simulink library "blind_cfr_lib"  (Simulink 8.7)
settings: Solver=ode45  StartTime=0.0  StopTime=10.0  RelTol=1e-3
undefined symbols (not defined in the file): AdvDSPBChannelOutDisplay, AdvDSPBDMemDisplay, cfr0_id, cfr_Params, clock_rate, dpoly, dspba_ChannelInVis, dspba_ChannelOutVis, dspba_internal_get_channel_ports, dspba_internal_get_demux_ports, evalAionMaskParam, iq_width, Iter0_Param, latency, primtype, PulsExtention, REG, REG_dut_id_addr, sample_rate, UseDontCare, value, win
libraries: DSPBAPrim x213, blind_cfr_lib x22, DSPBAControl x17, DSPBAModelBus x3, Pipereg_lib x2, CORDIC_lib x1
(part 1 of 3)
settings Model: Creator=nsafari  LastModifiedBy=5g

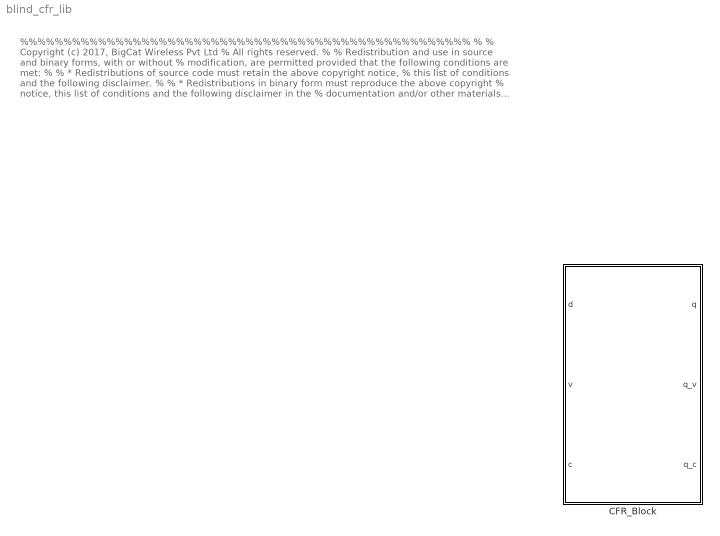
== system blind_cfr_lib ==
  note: %%%%%%%%%%%%%%%%%%%%%%%%%%%%%%%%%%%%%%%%%%%%%%%%%%%%
      |  %
      |  % Copyright (c) 2017, BigCat Wireless Pvt Ltd
      |  % All rights reserved.
      |  %
      |  % Redistribution and use in source and binary forms, with or without
      |  % modification, are permitted provided that the following conditions are met:
      |  %
      |  %     * Redistributions of source code must retain the above copyright notice,
      |  %       this list of conditions and the following disclaimer.
      |  %
      |  %     * Redistributions in binary form must reproduce the above copyright
      |  %       notice, this list of conditions and the following disclaimer in the
      |  %       documentation and/or other materials provided with the distribution.
      |  %
      |  %     * Neither the name of the copyright holder nor the names of its contributors
      |  %       may be used to endorse or promote products derived from this software
      |  %       without specific prior written permission.
      |  %
      |  %
      |  %
      |  % THIS SOFTWARE IS PROVIDED BY THE COPYRIGHT HOLDERS AND CONTRIBUTORS "AS IS"
      |  % AND ANY EXPRESS OR IMPLIED WARRANTIES, INCLUDING, BUT NOT LIMITED TO, THE
      |  % IMPLIED WARRANTIES OF MERCHANTABILITY AND FITNESS FOR A PARTICULAR PURPOSE ARE
      |  % DISCLAIMED. IN NO EVENT SHALL THE COPYRIGHT HOLDER OR CONTRIBUTORS BE LIABLE
      |  % FOR ANY DIRECT, INDIRECT, INCIDENTAL, SPECIAL, EXEMPLARY, OR CONSEQUENTIAL
      |  % DAMAGES (INCLUDING, BUT NOT LIMITED TO, PROCUREMENT OF SUBSTITUTE GOODS OR
      |  % SERVICES; LOSS OF USE, DATA, OR PROFITS; OR BUSINESS INTERRUPTION) HOWEVER
      |  % CAUSED AND ON ANY THEORY OF LIABILITY, WHETHER IN CONTRACT, STRICT LIABILITY,
      |  % OR TORT (INCLUDING NEGLIGENCE OR OTHERWISE) ARISING IN ANY WAY OUT OF THE USE
      |  % OF THIS SOFTWARE, EVEN IF ADVISED OF THE POSSIBILITY OF SUCH DAMAGE.
      |  %
      |   %%%%%%%%%%%%%%%%%%%%%%%%%%%%%%%%%%%%%%%%%%%%%%%%%%%
  CFR_Block : Subsystem  mask(Altera CFR Library Block){clk=clock_rate, sample_rate=sample_rate, block_id=cfr0_id, block_id_addr=REG_dut_id_addr, cfr_Params=cfr_Params, REG=REG, Pipeline_stages=0, ClockMargin=0}
      mask prompts: clk "System clock"; sample_rate "sample rate"; block_id "Unique ID of CFR"; block_id_addr "CFR ID address"; cfr_Params "CFR Configuration Structure"; REG "Register Map"
      mask help:
      | The block has the following parameters:
      |
      | "system clock" - the clock rate CFR module runs.
      |
      | "sample rate" - input signal sampling rate.
      |
      | "Folding Factor" - the number of folding for the module time-sharing;
      | It takes integer values between 1 and floor(system clock / sample rate).
      |
      | "Unique ID of CFR" is a unique numerical integer identifier for the CFR
      | block, this is used once the block is in a larger system to confirm the
      | correct block is being accessed.
      |
      | "CFR ID address" this is the relative address of the "Unique ID of CFR"
      | typically this is zero (at the CFR base address).
      |
      | "CFR Configuration Structure" - an array structure containing the
      | configuration of the CFR block. The length of this parameter specifies the
      | number of CFR core iterations instantiated.
      |
      | "Register Map" a structure containing the register map for CFR block.
      |
      | The settings of the above are exemplified in the setup script of the
      | altera_cfr example design.
      mask init:
      | %setup_cfr_block(iters, Iter_Params, REG, block_id, block_id_addr);
      mask Display:
      | fprintf('BLIND CFR');
      | port_label('input',1,'d');
      | port_label('input',2,'v');
      | port_label('input',3,'c');
      | port_label('output',1,'q');
      | port_label('output',2,'q_v');
      | port_label('output',3,'q_c');

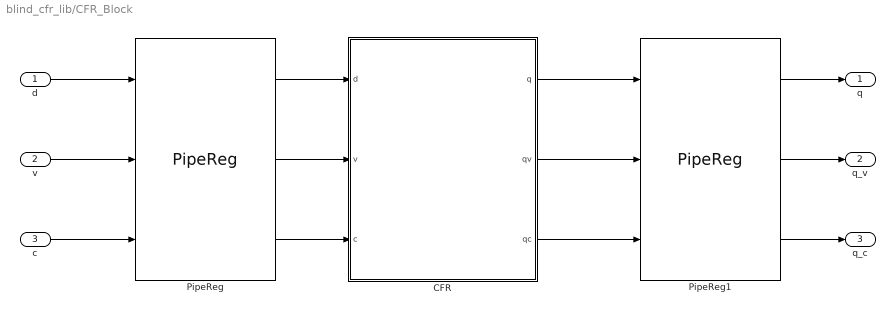
== system blind_cfr_lib/CFR_Block ==
  d : Inport
  v : Inport  Port=2
  c : Inport  Port=3
  CFR : Subsystem
  PipeReg : Pipereg_lib/PipeReg  NPipe=Pipeline_stages  Clock_Margin=ClockMargin
  PipeReg1 : Pipereg_lib/PipeReg  NPipe=Pipeline_stages  Clock_Margin=ClockMargin
  q : Outport
  q_v : Outport  Port=2
  q_c : Outport  Port=3
  wires:
  v/1 -> PipeReg/2
  c/1 -> PipeReg/3
  d/1 -> PipeReg/1
  PipeReg1/2 -> q_v/1
  PipeReg1/3 -> q_c/1
  PipeReg1/1 -> q/1
  PipeReg/2 -> CFR/2(v)
  PipeReg/3 -> CFR/3(c)
  PipeReg/1 -> CFR/1(d)
  CFR/1(q) -> PipeReg1/1
  CFR/2(qv) -> PipeReg1/2
  CFR/3(qc) -> PipeReg1/3

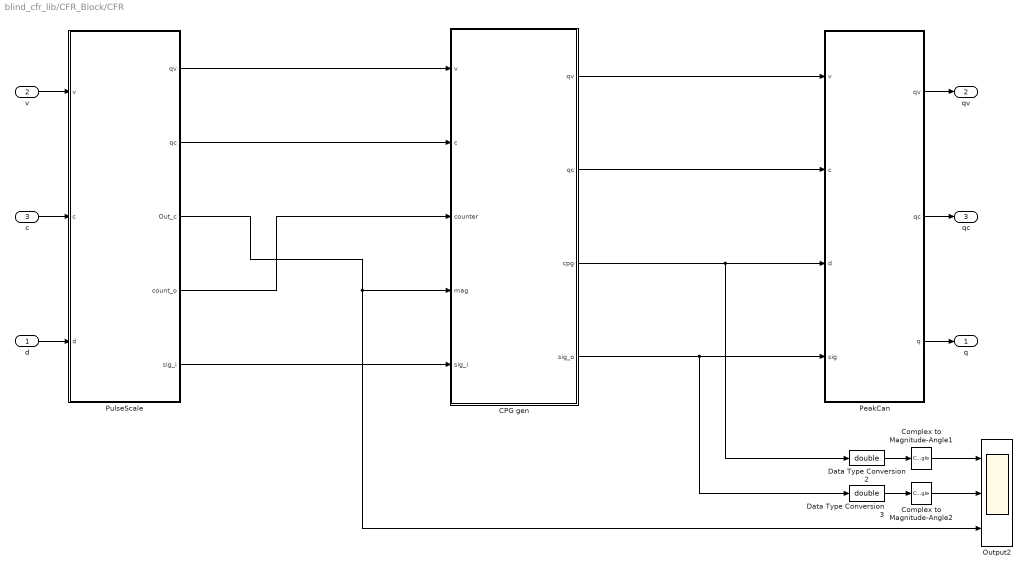
== system blind_cfr_lib/CFR_Block/CFR ==
  d : Inport
  v : Inport  Port=2
  c : Inport  Port=3
  CPG gen : Subsystem
  Complex to Magnitude-Angle1 : ComplexToMagnitudeAngle  Output=Magnitude
  Complex to Magnitude-Angle2 : ComplexToMagnitudeAngle  Output=Magnitude
  Data Type Conversion2 : DataTypeConversion  OutDataTypeStr=double
  Data Type Conversion3 : DataTypeConversion  OutDataTypeStr=double
  Output2 : Scope  NumInputPorts=3
  PeakCan : Subsystem
  PulseScale : Subsystem
  q : Outport
  qv : Outport  Port=2
  qc : Outport  Port=3
  wires:
  v/1 -> PulseScale/1(v)
  c/1 -> PulseScale/2(c)
  PeakCan/1(qv) -> qv/1
  PeakCan/2(qc) -> qc/1
  PeakCan/3(q) -> q/1
  CPG gen/3(cpg) -> Data Type Conversion2/1, PeakCan/3(d)
  CPG gen/4(sig_o) -> Data Type Conversion3/1, PeakCan/4(sig)
  CPG gen/1(qv) -> PeakCan/1(v)
  CPG gen/2(qc) -> PeakCan/2(c)
  PulseScale/1(qv) -> CPG gen/1(v)
  PulseScale/2(qc) -> CPG gen/2(c)
  PulseScale/3(Out_c) -> Output2/3, CPG gen/4(mag)
  PulseScale/4(count_o) -> CPG gen/3(counter)
  Data Type Conversion2/1 -> Complex to Magnitude-Angle1/1
  Complex to Magnitude-Angle1/1 -> Output2/1
  Data Type Conversion3/1 -> Complex to Magnitude-Angle2/1
  Complex to Magnitude-Angle2/1 -> Output2/2
  d/1 -> PulseScale/3(d)
  PulseScale/5(sig_i) -> CPG gen/5(sig_i)

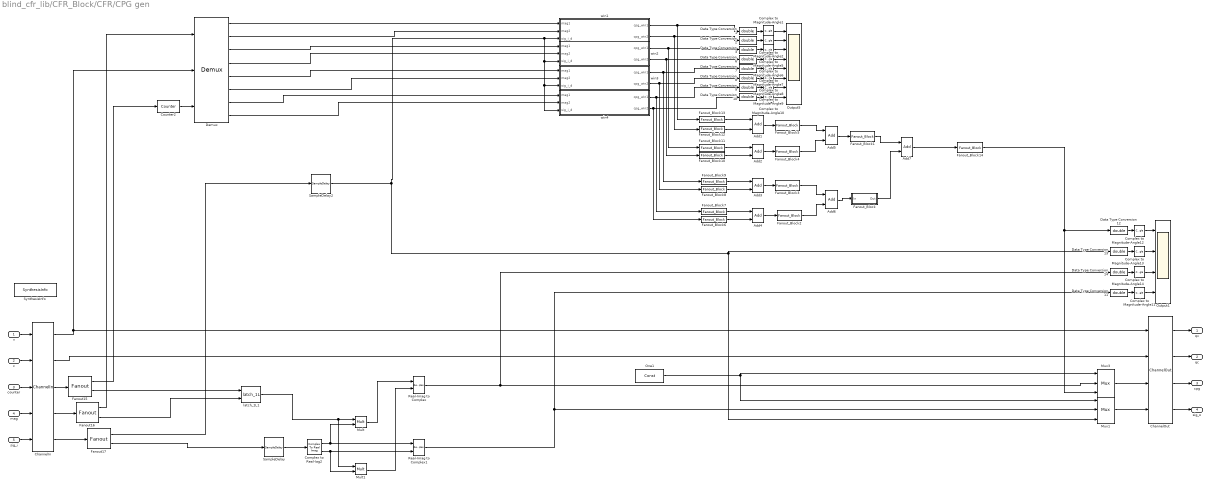
== system blind_cfr_lib/CFR_Block/CFR/CPG gen ==
  v : Inport
  c : Inport  Port=2
  counter : Inport  Port=3
  mag : Inport  Port=4
  sig_i : Inport  Port=5
  Add{1..7} (7 alike) : DSPBAPrim/Add  primtype=add  nInputs=evalAionMaskParam(gcb,'value',1)  nOutputs=1  omode=Inherit via internal rule with word growth  otype=sfix(16)  scale=2^-15  rndmethod=Unbiased  factor=1  satmethod=Symmetric  shift_vec=[0 1 2 -1]  value=2  inPortNames=[' '; ' ';]  outPortNames=[' ']  dspbaimage=dspba_prim.jpg  text=fprintf('+');  style=Optimised  visibilities=1032+2^17+2^18+2^19  genFPC=off  floatRounding=correct  advOptions=[]  version=20130821
  ChannelIn : DSPBAPrim/ChannelIn  primtype=channelin  nInputs=dspba_internal_get_channel_ports(gcb)  nOutputs=dspba_internal_get_channel_ports(gcb)  omode=Inherit via internal rule  otype=sfix(16)  scale=2^-15  rndmethod=Unbiased  factor=1  satmethod=Symmetric  shift_vec=[0 1 2 -1]  value=3  inPortNames=['v'; 'c'; '0'; '1'; '2'; '3'; '4'; '5'; '6'; '7'; '8'; '9'; 'A'; 'B'; 'D'; 'E'; 'F'; 'G'; 'H'; 'I'; 'J'; 'K'; 'L'; 'M'; 'N'; 'O'; 'P'; 'Q'; 'R'; 'S'; 'T'; 'U'; 'W'; 'X'; 'Y'; 'Z']  outPortNames=['v'; 'c'; '0'; '1'; '2'; '3'; '4'; '5'; '6'; '7'; '8'; '9'; 'A'; 'B'; 'D'; 'E'; 'F'; 'G'; 'H'; 'I'; 'J'; 'K'; 'L'; 'M'; 'N'; 'O'; 'P'; 'Q'; 'R'; 'S'; 'T'; 'U'; 'W'; 'X'; 'Y'; 'Z']  dspbaimage=dspba_prim.jpg  text=fprintf('In');  style=Optimised  dataSignals=3  foldingEnabled=off  channels=1  sampleRate=200  packetBeginPresent=off  packetBeginEnabled=off  visibilities=dspba_ChannelInVis(gcb)  latencyCorrection=0  version=20141013
  ChannelOut : DSPBAPrim/ChannelOut  primtype=channelout  nInputs=dspba_internal_get_channel_ports(gcb)  nOutputs=dspba_internal_get_channel_ports(gcb)  omode=Inherit via internal rule  otype=sfix(16)  scale=2^-15  rndmethod=Unbiased  factor=1  satmethod=Symmetric  shift_vec=[0 1 2 -1]  value=2  inPortNames=['v'; 'c'; '0'; '1'; '2'; '3'; '4'; '5'; '6'; '7'; '8'; '9'; 'A'; 'B'; 'D'; 'E'; 'F'; 'G'; 'H'; 'I'; 'J'; 'K'; 'L'; 'M'; 'N'; 'O'; 'P'; 'Q'; 'R'; 'S'; 'T'; 'U'; 'W'; 'X'; 'Y'; 'Z']  outPortNames=['v'; 'c'; '0'; '1'; '2'; '3'; '4'; '5'; '6'; '7'; '8'; '9'; 'A'; 'B'; 'D'; 'E'; 'F'; 'G'; 'H'; 'I'; 'J'; 'K'; 'L'; 'M'; 'N'; 'O'; 'P'; 'Q'; 'R'; 'S'; 'T'; 'U'; 'W'; 'X'; 'Y'; 'Z']  dspbaimage=dspba_prim.jpg  text=fprintf('Out%s', AdvDSPBChannelOutDisplay(latency));  style=Optimised  dataSignals=2  foldingEnabled=off  channels=1  sampleRate=200  packetBeginPresent=off  packetBeginEnabled=off  visibilities=dspba_ChannelOutVis(gcb)  latency=16  latencyCorrection=0  version=20141013
  Complex to Magnitude-Angle{1..2,5..14} (12 alike) : ComplexToMagnitudeAngle  Output=Magnitude
  Complex to Real-Iag2 : ComplexToRealImag
  Counter2 : DSPBAPrim/Counter  primtype=counter  nInputs=1  nOutputs=1  omode=Inherit via internal rule  otype=ufix(16)  scale=2^-0  rndmethod=Unbiased  factor=1  satmethod=Symmetric  shift_vec=[0 1 2 -1]  value=[0 8 1]  inPortNames=[' '; ' ';]  outPortNames=[' ']  dspbaimage=dspba_prim.jpg  text=fprintf('counter\n[%d %d %d]', value(1), value(2), value(3));  style=Optimised  visibilities=8 + 1024  version=20090407
  Data Type Conversion{1..3,6..14} (12 alike) : DataTypeConversion  OutDataTypeStr=double
  Demux : DSPBAPrim/Demux  primtype=demux  nInputs=3  nOutputs=dspba_internal_get_demux_ports(gcb)  omode=Inherit via internal rule  otype=sfix(16)  scale=2^-15  rndmethod=Unbiased  factor=1  satmethod=Symmetric  shift_vec=[0 1 2 3 4 5 6 7]  value=8  inPortNames=['q'; 'v'; 'c']  outPortNames=['c0'; 'c1']  dspbaimage=dspba_prim.jpg  text=fprintf('demux');  style=Optimised  visibilities=1536  version=20100120
  Fanout15 : DSPBAPrim/Fanout  primtype=fanout  nInputs=1  nOutputs=evalAionMaskParam(gcb,'value',1)  omode=Inherit via internal rule  otype=sfix(16)  scale=2^-15  rndmethod=Unbiased  factor=1  satmethod=Symmetric  shift_vec=[0 1 2 -1]  value=2  inPortNames=[' '; ' ';]  outPortNames=[' ']  dspbaimage=dspba_prim.jpg  text=fprintf('fanout')  style=Optimised  visibilities=2^10+2^18  version=20150501  uninit=off
  Fanout16 : DSPBAPrim/Fanout  primtype=fanout  nInputs=1  nOutputs=evalAionMaskParam(gcb,'value',1)  omode=Inherit via internal rule  otype=sfix(16)  scale=2^-15  rndmethod=Unbiased  factor=1  satmethod=Symmetric  shift_vec=[0 1 2 -1]  value=2  inPortNames=[' '; ' ';]  outPortNames=[' ']  dspbaimage=dspba_prim.jpg  text=fprintf('fanout')  style=Optimised  visibilities=2^10+2^18  version=20150501  uninit=off
  Fanout17 : DSPBAPrim/Fanout  primtype=fanout  nInputs=1  nOutputs=evalAionMaskParam(gcb,'value',1)  omode=Inherit via internal rule  otype=sfix(16)  scale=2^-15  rndmethod=Unbiased  factor=1  satmethod=Symmetric  shift_vec=[0 1 2 -1]  value=2  inPortNames=[' '; ' ';]  outPortNames=[' ']  dspbaimage=dspba_prim.jpg  text=fprintf('fanout')  style=Optimised  visibilities=2^10+2^18  version=20150501  uninit=off
  Fanout_Block : Subsystem
  Fanout_Block{1..14} (14 alike) : blind_cfr_lib/CFR_Block/CFR/CPG gen/Fanout_Block
  Mult : DSPBAPrim/Mult  primtype=mult  nInputs=2  nOutputs=1  omode=Inherit via internal rule  otype=sfix(16)  scale=2^-15  rndmethod=Unbiased  factor=1  satmethod=Symmetric  shift_vec=[0 1 2 -1]  value=0  inPortNames=[' '; ' ';]  outPortNames=[' ']  dspbaimage=dspba_prim.jpg  text=fprintf('X');  style=Optimised  visibilities=8+2^18+2^19  floatPrecision=float32_m23  floatRounding=correct  advOptions=[]  version=20130115
  Mult1 : DSPBAPrim/Mult  primtype=mult  nInputs=2  nOutputs=1  omode=Inherit via internal rule  otype=sfix(16)  scale=2^-15  rndmethod=Unbiased  factor=1  satmethod=Symmetric  shift_vec=[0 1 2 -1]  value=0  inPortNames=[' '; ' ';]  outPortNames=[' ']  dspbaimage=dspba_prim.jpg  text=fprintf('X');  style=Optimised  visibilities=8+2^18+2^19  floatPrecision=float32_m23  floatRounding=correct  advOptions=[]  version=20130115
  Mux1 : DSPBAPrim/Mux  primtype=mux  nInputs=evalAionMaskParam(gcb,'value',1)+1  nOutputs=1  omode=Inherit via internal rule  otype=sfix(16)  scale=2^-15  rndmethod=Unbiased  factor=1  satmethod=Symmetric  shift_vec=[0 1 2 -1]  value=2  inPortNames=['s'; 'd0'; 'd1'; 'd2'; 'd3'; 'd4'; 'd5'; 'd6'; 'd7'; 'd8'; 'd9';]  outPortNames=[' ']  dspbaimage=dspba_prim.jpg  text=fprintf('%s', primtype);  style=Optimised  visibilities=1032  version=20131025
  Mux3 : DSPBAPrim/Mux  primtype=mux  nInputs=evalAionMaskParam(gcb,'value',1)+1  nOutputs=1  omode=Inherit via internal rule  otype=sfix(16)  scale=2^-15  rndmethod=Unbiased  factor=1  satmethod=Symmetric  shift_vec=[0 1 2 -1]  value=2  inPortNames=['s'; 'd0'; 'd1'; 'd2'; 'd3'; 'd4'; 'd5'; 'd6'; 'd7'; 'd8'; 'd9';]  outPortNames=[' ']  dspbaimage=dspba_prim.jpg  text=fprintf('%s', primtype);  style=Optimised  visibilities=1032  version=20131025
  One1 : DSPBAPrim/Const  primtype=const  nInputs=0  nOutputs=1  omode=boolean  otype=uint(1)  scale=2^0  rndmethod=Unbiased  factor=1  satmethod=Symmetric  shift_vec=[0 1 2 -1]  value=win_enable  inPortNames=['+'; '+';]  outPortNames=[' ']  dspbaimage=dspba_prim.jpg  text=fprintf('%s', num2str(value));  style=Optimised  visibilities=8 + 1024  floatPrecision=float32_m23  version=20120820
  Output1 : Scope  NumInputPorts=4
  Output5 : Scope  NumInputPorts=8
  Real-Imag to Complex : RealImagToComplex
  Real-Imag to Complex1 : RealImagToComplex
  SampleDelay : DSPBAPrim/SampleDelay  primtype=sampdelay  nInputs=1  nOutputs=1  omode=Inherit via internal rule  otype=uint(16)  scale=2^-0  rndmethod=Unbiased  factor=1  satmethod=Symmetric  shift_vec=[0 1 2 -1]  value=Iter0_Param.pulseLen  inPortNames=[' '; ' ';]  outPortNames=[' ']  dspbaimage=dspba_prim.jpg  text=dpoly(1, eye(1,value+1), 'z')  style=Optimised  visibilities=8 + 1024  flexible=off  slackgroup=0  augmented=0  version=20090407  advOptions=[]
  SampleDelay2 : DSPBAPrim/SampleDelay  primtype=sampdelay  nInputs=1  nOutputs=1  omode=Inherit via internal rule  otype=uint(16)  scale=2^-0  rndmethod=Unbiased  factor=1  satmethod=Symmetric  shift_vec=[0 1 2 -1]  value=Iter0_Param.pulseLen + PulsExtention  inPortNames=[' '; ' ';]  outPortNames=[' ']  dspbaimage=dspba_prim.jpg  text=dpoly(1, eye(1,value+1), 'z')  style=Optimised  visibilities=8 + 1024  flexible=off  slackgroup=0  augmented=0  version=20090407  advOptions=[]
  SynthesisInfo : DSPBAPrim/SynthesisInfo  primtype=synthinfo  nInputs=0  nOutputs=0  omode=Inherit via internal rule  otype=sfix(16)  scale=2^-15  rndmethod=Truncate  factor=1  satmethod=Symmetric  shift_vec=[0 1 2 -1]  value=99  inPortNames=[' '; ' ';]  outPortNames=[' ']  dspbaimage=dspba_prim.jpg  text=fprintf('Style=%s', style);  style=Scheduled  visibilities=32768  constraintInUse=off  constraintRelation=>  constraintLimit=50  bitAccurate=off  version=20150220
  latch_1L1 : DSPBAControl/latch_1L
  win1 : Subsystem
  win2 : Subsystem
  win3 : Subsystem
  win4 : Subsystem
  qv : Outport
  qc : Outport  Port=2
  cpg : Outport  Port=3
  sig_o : Outport  Port=4
  wires:
  Mult/1 -> Real-Imag to Complex/1
  Mult1/1 -> Real-Imag to Complex/2
  Complex to Real-Iag2/2 -> Mult1/2, Real-Imag to Complex1/2
  v/1 -> ChannelIn/1
  c/1 -> ChannelIn/2
  ChannelIn/2 -> ChannelOut/2
  Real-Imag to Complex/1 -> Data Type Conversion14/1, Mux3/2
  ChannelOut/1 -> qv/1
  ChannelOut/2 -> qc/1
  counter/1 -> ChannelIn/3
  mag/1 -> ChannelIn/4
  ChannelOut/3 -> cpg/1
  ChannelOut/4 -> sig_o/1
  Complex to Real-Iag2/1 -> Mult/2, Real-Imag to Complex1/1
  Real-Imag to Complex1/1 -> Mux1/2, Data Type Conversion11/1
  sig_i/1 -> ChannelIn/5
  latch_1L1/1 -> Mult1/1, Mult/1
  ChannelIn/1 -> Demux/2, ChannelOut/1
  SampleDelay/1 -> Complex to Real-Iag2/1
  Counter2/1 -> Demux/3
  Data Type Conversion1/1 -> Complex to Magnitude-Angle1/1
  Complex to Magnitude-Angle1/1 -> Output5/1
  Data Type Conversion2/1 -> Complex to Magnitude-Angle2/1
  Complex to Magnitude-Angle2/1 -> Output5/2
  Demux/1 -> win1/1(mag1)
  Demux/2 -> win1/2(mag2)
  SampleDelay2/1 -> win1/3(sig_i_d), win2/3(sig_i_d), win4/3(sig_i_d), win3/3(sig_i_d), Mux1/3, Data Type Conversion13/1
  win1/1(cpg_win1) -> Fanout_Block13/1, Data Type Conversion1/1
  win1/2(cpg_win2) -> Fanout_Block12/1, Data Type Conversion2/1
  Demux/3 -> win2/1(mag1)
  Demux/4 -> win2/2(mag2)
  Data Type Conversion3/1 -> Complex to Magnitude-Angle5/1
  Complex to Magnitude-Angle5/1 -> Output5/3
  Data Type Conversion6/1 -> Complex to Magnitude-Angle6/1
  Complex to Magnitude-Angle6/1 -> Output5/4
  Data Type Conversion7/1 -> Complex to Magnitude-Angle7/1
  Complex to Magnitude-Angle7/1 -> Output5/5
  Data Type Conversion8/1 -> Complex to Magnitude-Angle8/1
  Complex to Magnitude-Angle8/1 -> Output5/6
  Data Type Conversion9/1 -> Complex to Magnitude-Angle9/1
  Complex to Magnitude-Angle9/1 -> Output5/7
  Data Type Conversion10/1 -> Complex to Magnitude-Angle10/1
  Complex to Magnitude-Angle10/1 -> Output5/8
  win2/1(cpg_win1) -> Fanout_Block11/1, Data Type Conversion3/1
  win2/2(cpg_win2) -> Fanout_Block10/1, Data Type Conversion6/1
  Demux/5 -> win3/1(mag1)
  Demux/6 -> win3/2(mag2)
  Demux/7 -> win4/1(mag1)
  Demux/8 -> win4/2(mag2)
  win3/1(cpg_win1) -> Fanout_Block9/1, Data Type Conversion7/1
  win3/2(cpg_win2) -> Fanout_Block8/1, Data Type Conversion8/1
  win4/1(cpg_win1) -> Fanout_Block7/1, Data Type Conversion9/1
  win4/2(cpg_win2) -> Fanout_Block6/1, Data Type Conversion10/1
  Data Type Conversion12/1 -> Complex to Magnitude-Angle12/1
  Complex to Magnitude-Angle12/1 -> Output1/1
  Data Type Conversion13/1 -> Complex to Magnitude-Angle13/1
  Complex to Magnitude-Angle13/1 -> Output1/2
  Data Type Conversion14/1 -> Complex to Magnitude-Angle14/1
  Complex to Magnitude-Angle14/1 -> Output1/3
  Data Type Conversion11/1 -> Complex to Magnitude-Angle11/1
  Complex to Magnitude-Angle11/1 -> Output1/4
  One1/1 -> Mux1/1, Mux3/1
  Mux3/1 -> ChannelOut/3
  Mux1/1 -> ChannelOut/4
  Fanout_Block13/1 -> Add1/1
  Fanout_Block12/1 -> Add1/2
  Fanout_Block14/1 -> Data Type Conversion12/1, Mux3/3
  Fanout_Block11/1 -> Add2/1
  Fanout_Block10/1 -> Add2/2
  Fanout_Block9/1 -> Add3/1
  Fanout_Block8/1 -> Add3/2
  Fanout_Block7/1 -> Add4/1
  Add1/1 -> Fanout_Block5/1
  Add4/1 -> Fanout_Block2/1
  Add3/1 -> Fanout_Block3/1
  Add2/1 -> Fanout_Block4/1
  Fanout_Block5/1 -> Add5/1
  Fanout_Block4/1 -> Add5/2
  Fanout_Block3/1 -> Add6/1
  Fanout_Block2/1 -> Add6/2
  Add5/1 -> Fanout_Block1/1
  Fanout_Block1/1 -> Add7/1
  Add7/1 -> Fanout_Block14/1
  ChannelIn/3 -> Fanout15/1
  Fanout15/2 -> latch_1L1/1
  Fanout15/1 -> Counter2/1
  ChannelIn/4 -> Fanout16/1
  Fanout16/1 -> Demux/1
  Fanout16/2 -> latch_1L1/2
  ChannelIn/5 -> Fanout17/1
  Fanout17/2 -> SampleDelay/1
  Fanout17/1 -> SampleDelay2/1
  Add6/1 -> Fanout_Block/1(In)
  Fanout_Block/1(Out) -> Add7/2
  Fanout_Block6/1 -> Add4/2

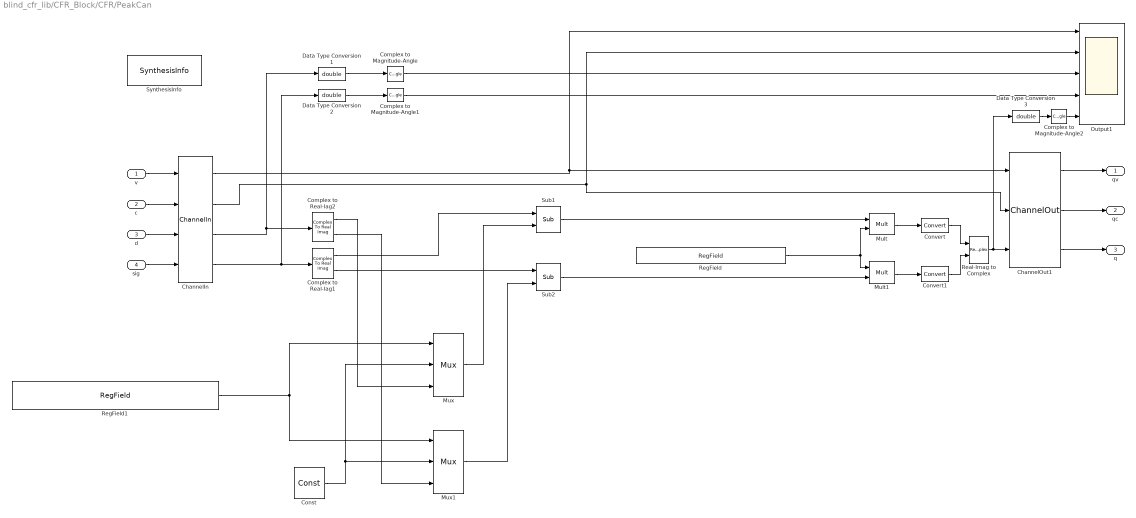
== system blind_cfr_lib/CFR_Block/CFR/PeakCan ==
  v : Inport
  c : Inport  Port=2
  d : Inport  Port=3
  sig : Inport  Port=4
  ChannelIn : DSPBAPrim/ChannelIn  primtype=channelin  nInputs=dspba_internal_get_channel_ports(gcb)  nOutputs=dspba_internal_get_channel_ports(gcb)  omode=Inherit via internal rule  otype=sfix(16)  scale=2^-15  rndmethod=Unbiased  factor=1  satmethod=Symmetric  shift_vec=[0 1 2 -1]  value=2  inPortNames=['v'; 'c'; '0'; '1'; '2'; '3'; '4'; '5'; '6'; '7'; '8'; '9'; 'A'; 'B'; 'D'; 'E'; 'F'; 'G'; 'H'; 'I'; 'J'; 'K'; 'L'; 'M'; 'N'; 'O'; 'P'; 'Q'; 'R'; 'S'; 'T'; 'U'; 'W'; 'X'; 'Y'; 'Z']  outPortNames=['v'; 'c'; '0'; '1'; '2'; '3'; '4'; '5'; '6'; '7'; '8'; '9'; 'A'; 'B'; 'D'; 'E'; 'F'; 'G'; 'H'; 'I'; 'J'; 'K'; 'L'; 'M'; 'N'; 'O'; 'P'; 'Q'; 'R'; 'S'; 'T'; 'U'; 'W'; 'X'; 'Y'; 'Z']  dspbaimage=dspba_prim.jpg  text=fprintf('In');  style=Optimised  dataSignals=2  foldingEnabled=off  channels=1  sampleRate=200  packetBeginPresent=off  packetBeginEnabled=off  visibilities=dspba_ChannelInVis(gcb)  latencyCorrection=0  version=20141013
  ChannelOut1 : DSPBAPrim/ChannelOut  primtype=channelout  nInputs=dspba_internal_get_channel_ports(gcb)  nOutputs=dspba_internal_get_channel_ports(gcb)  omode=Inherit via internal rule  otype=sfix(16)  scale=2^-15  rndmethod=Unbiased  factor=1  satmethod=Symmetric  shift_vec=[0 1 2 -1]  value=1  inPortNames=['v'; 'c'; '0'; '1'; '2'; '3'; '4'; '5'; '6'; '7'; '8'; '9'; 'A'; 'B'; 'D'; 'E'; 'F'; 'G'; 'H'; 'I'; 'J'; 'K'; 'L'; 'M'; 'N'; 'O'; 'P'; 'Q'; 'R'; 'S'; 'T'; 'U'; 'W'; 'X'; 'Y'; 'Z']  outPortNames=['v'; 'c'; '0'; '1'; '2'; '3'; '4'; '5'; '6'; '7'; '8'; '9'; 'A'; 'B'; 'D'; 'E'; 'F'; 'G'; 'H'; 'I'; 'J'; 'K'; 'L'; 'M'; 'N'; 'O'; 'P'; 'Q'; 'R'; 'S'; 'T'; 'U'; 'W'; 'X'; 'Y'; 'Z']  dspbaimage=dspba_prim.jpg  text=fprintf('Out%s', AdvDSPBChannelOutDisplay(latency));  style=Optimised  dataSignals=1  foldingEnabled=off  channels=1  sampleRate=200  packetBeginPresent=off  packetBeginEnabled=off  visibilities=dspba_ChannelOutVis(gcb)  latency=12  latencyCorrection=0  version=20141013
  Complex to Magnitude-Angle : ComplexToMagnitudeAngle  Output=Magnitude
  Complex to Magnitude-Angle1 : ComplexToMagnitudeAngle  Output=Magnitude
  Complex to Magnitude-Angle2 : ComplexToMagnitudeAngle  Output=Magnitude
  Complex to Real-Iag1 : ComplexToRealImag
  Complex to Real-Iag2 : ComplexToRealImag
  Const : DSPBAPrim/Const  primtype=const  nInputs=0  nOutputs=1  omode=Inherit via internal rule  otype=sfix(16)  scale=2^-15  rndmethod=Unbiased  factor=1  satmethod=Symmetric  shift_vec=[0 1 2 -1]  value=0  inPortNames=['+'; '+';]  outPortNames=[' ']  dspbaimage=dspba_prim.jpg  text=fprintf('%s', num2str(value));  style=Optimised  visibilities=8 + 1024  floatPrecision=float32_m23  version=20120820
  Convert : DSPBAPrim/Convert  primtype=convert  nInputs=1  nOutputs=1  omode=Specify via dialog  otype=sfix(16)  scale=2^-15  rndmethod=Unbiased  factor=1  satmethod=None  shift_vec=[0 1 2 -1]  value=round([0:255]/17)  inPortNames=[' '; ' ';]  outPortNames=[' '; 'c']  dspbaimage=dspba_prim.jpg  text=fprintf('convert');  style=Optimised  visibilities=8+64+256+2^17  clipdetect=off  floatPrecision=float32_m23  advOptions=[]  version=20130211
  Convert1 : DSPBAPrim/Convert  primtype=convert  nInputs=1  nOutputs=1  omode=Specify via dialog  otype=sfix(16)  scale=2^-15  rndmethod=Unbiased  factor=1  satmethod=None  shift_vec=[0 1 2 -1]  value=round([0:255]/17)  inPortNames=[' '; ' ';]  outPortNames=[' '; 'c']  dspbaimage=dspba_prim.jpg  text=fprintf('convert');  style=Optimised  visibilities=8+64+256+2^17  clipdetect=off  floatPrecision=float32_m23  advOptions=[]  version=20130211
  Data Type Conversion1 : DataTypeConversion  OutDataTypeStr=double
  Data Type Conversion2 : DataTypeConversion  OutDataTypeStr=double
  Data Type Conversion3 : DataTypeConversion  OutDataTypeStr=double
  Mult : DSPBAPrim/Mult  primtype=mult  nInputs=2  nOutputs=1  omode=Inherit via internal rule  otype=sfix(16)  scale=2^-15  rndmethod=Unbiased  factor=1  satmethod=Symmetric  shift_vec=[0 1 2 -1]  value=0  inPortNames=[' '; ' ';]  outPortNames=[' ']  dspbaimage=dspba_prim.jpg  text=fprintf('X');  style=Optimised  visibilities=8+2^18+2^19  floatPrecision=float32_m23  floatRounding=correct  advOptions=[]  version=20130115
  Mult1 : DSPBAPrim/Mult  primtype=mult  nInputs=2  nOutputs=1  omode=Inherit via internal rule  otype=sfix(16)  scale=2^-15  rndmethod=Unbiased  factor=1  satmethod=Symmetric  shift_vec=[0 1 2 -1]  value=0  inPortNames=[' '; ' ';]  outPortNames=[' ']  dspbaimage=dspba_prim.jpg  text=fprintf('X');  style=Optimised  visibilities=8+2^18+2^19  floatPrecision=float32_m23  floatRounding=correct  advOptions=[]  version=20130115
  Mux : DSPBAPrim/Mux  primtype=mux  nInputs=evalAionMaskParam(gcb,'value',1)+1  nOutputs=1  omode=Inherit via internal rule  otype=sfix(16)  scale=2^-15  rndmethod=Unbiased  factor=1  satmethod=Symmetric  shift_vec=[0 1 2 -1]  value=2  inPortNames=['s '; 'd0'; 'd1'; 'd2'; 'd3'; 'd4'; 'd5'; 'd6'; 'd7'; 'd8'; 'd9';]  outPortNames=[' ']  dspbaimage=dspba_prim.jpg  text=fprintf('%s', primtype);  style=Optimised  visibilities=1032  version=20131025
  Mux1 : DSPBAPrim/Mux  primtype=mux  nInputs=evalAionMaskParam(gcb,'value',1)+1  nOutputs=1  omode=Inherit via internal rule  otype=sfix(16)  scale=2^-15  rndmethod=Unbiased  factor=1  satmethod=Symmetric  shift_vec=[0 1 2 -1]  value=2  inPortNames=['s '; 'd0'; 'd1'; 'd2'; 'd3'; 'd4'; 'd5'; 'd6'; 'd7'; 'd8'; 'd9';]  outPortNames=[' ']  dspbaimage=dspba_prim.jpg  text=fprintf('%s', primtype);  style=Optimised  visibilities=1032  version=20131025
  Output1 : Scope  NumInputPorts=5
  Real-Imag to Complex : RealImagToComplex
  RegField : DSPBAModelBus/RegField  reg_name=cfr_Params.BaseAddr + REG.Scaling  reg_rwmode=Read/Write  reg_msb=15  reg_lsb=0  reg_mode=Specify via dialog  reg_type=ufix(16)  reg_scale=2^-14  reg_init=cfr_Params.Scaling  reg_desc=Scaling value  reg_modal=off  reg_desc0=0  reg_desc1=0  reg_desc2=0  reg_desc3=0  reg_desc4=0  reg_desc5=0  reg_desc6=0  reg_desc7=0  SampleTime=1  version=20090407
  RegField1 : DSPBAModelBus/RegField  reg_name=cfr_Params.BaseAddr + REG.Enable  reg_rwmode=Read/Write  reg_msb=0  reg_lsb=0  reg_mode=Specify via dialog  reg_type=ufix(1)  reg_scale=2^0  reg_init=cfr_Params.Enable  reg_desc=Enable CFR  reg_modal=off  reg_desc0=0  reg_desc1=0  reg_desc2=0  reg_desc3=0  reg_desc4=0  reg_desc5=0  reg_desc6=0  reg_desc7=0  SampleTime=1  version=20090407
  Sub1 : DSPBAPrim/Sub  primtype=sub  nInputs=2  nOutputs=1  omode=Inherit via internal rule  otype=sfix(16)  scale=2^-15  rndmethod=Unbiased  factor=1  satmethod=Symmetric  shift_vec=[0 1 2 -1]  value=0  inPortNames=['+'; '-';]  outPortNames=[' ']  dspbaimage=dspba_prim.jpg  text=fprintf('-');  style=Optimised  visibilities=8  floatRounding=correct  advOptions=[]  version=20130115
  Sub2 : DSPBAPrim/Sub  primtype=sub  nInputs=2  nOutputs=1  omode=Inherit via internal rule  otype=sfix(16)  scale=2^-15  rndmethod=Unbiased  factor=1  satmethod=Symmetric  shift_vec=[0 1 2 -1]  value=0  inPortNames=['+'; '-';]  outPortNames=[' ']  dspbaimage=dspba_prim.jpg  text=fprintf('-');  style=Optimised  visibilities=8  floatRounding=correct  advOptions=[]  version=20130115
  SynthesisInfo : DSPBAPrim/SynthesisInfo  primtype=synthinfo  nInputs=0  nOutputs=0  omode=Inherit via internal rule  otype=sfix(16)  scale=2^-15  rndmethod=Truncate  factor=1  satmethod=Symmetric  shift_vec=[0 1 2 -1]  value=99  inPortNames=[' '; ' ';]  outPortNames=[' ']  dspbaimage=dspba_prim.jpg  text=fprintf('Style=%s', style);  style=Scheduled  visibilities=32768  constraintInUse=off  constraintRelation=>  constraintLimit=20  bitAccurate=off  version=20150220
  qv : Outport
  qc : Outport  Port=2
  q : Outport  Port=3
  wires:
  Data Type Conversion1/1 -> Complex to Magnitude-Angle/1
  Complex to Magnitude-Angle/1 -> Output1/3
  ChannelIn/3 -> Data Type Conversion1/1, Complex to Real-Iag2/1
  Data Type Conversion2/1 -> Complex to Magnitude-Angle1/1
  Complex to Magnitude-Angle1/1 -> Output1/4
  Real-Imag to Complex/1 -> Data Type Conversion3/1, ChannelOut1/3
  Complex to Real-Iag1/1 -> Sub1/1
  Complex to Real-Iag1/2 -> Sub2/1
  ChannelIn/1 -> Output1/1, ChannelOut1/1
  ChannelIn/2 -> ChannelOut1/2, Output1/2
  v/1 -> ChannelIn/1
  d/1 -> ChannelIn/3
  c/1 -> ChannelIn/2
  sig/1 -> ChannelIn/4
  ChannelOut1/1 -> qv/1
  ChannelOut1/2 -> qc/1
  ChannelOut1/3 -> q/1
  ChannelIn/4 -> Complex to Real-Iag1/1, Data Type Conversion2/1
  RegField/1 -> Mult/2, Mult1/1
  Mult/1 -> Convert/1
  Mult1/1 -> Convert1/1
  Sub1/1 -> Mult/1
  Sub2/1 -> Mult1/2
  Convert/1 -> Real-Imag to Complex/1
  Convert1/1 -> Real-Imag to Complex/2
  Data Type Conversion3/1 -> Complex to Magnitude-Angle2/1
  Complex to Magnitude-Angle2/1 -> Output1/5
  RegField1/1 -> Mux/1, Mux1/1
  Complex to Real-Iag2/1 -> Mux/3
  Complex to Real-Iag2/2 -> Mux1/3
  Mux/1 -> Sub1/2
  Mux1/1 -> Sub2/2
  Const/1 -> Mux/2, Mux1/2

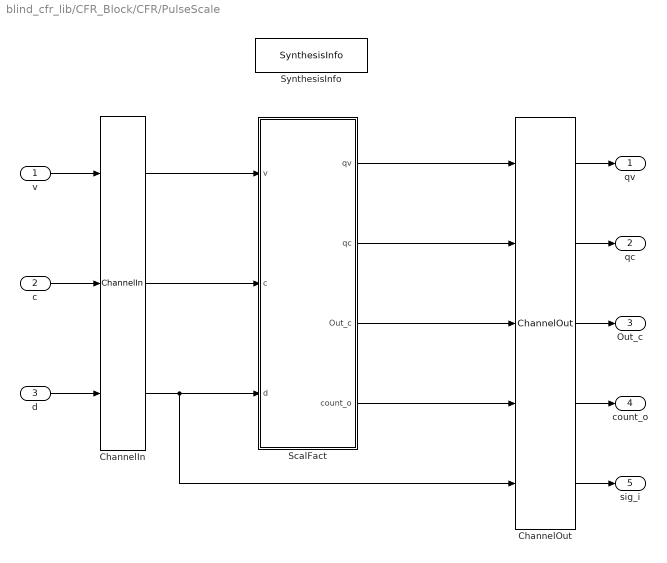
== system blind_cfr_lib/CFR_Block/CFR/PulseScale ==
  v : Inport
  c : Inport  Port=2
  d : Inport  Port=3
  ChannelIn : DSPBAPrim/ChannelIn  primtype=channelin  nInputs=dspba_internal_get_channel_ports(gcb)  nOutputs=dspba_internal_get_channel_ports(gcb)  omode=Inherit via internal rule  otype=sfix(16)  scale=2^-15  rndmethod=Unbiased  factor=1  satmethod=Symmetric  shift_vec=[0 1 2 -1]  value=1  inPortNames=['v'; 'c'; '0'; '1'; '2'; '3'; '4'; '5'; '6'; '7'; '8'; '9'; 'A'; 'B'; 'D'; 'E'; 'F'; 'G'; 'H'; 'I'; 'J'; 'K'; 'L'; 'M'; 'N'; 'O'; 'P'; 'Q'; 'R'; 'S'; 'T'; 'U'; 'W'; 'X'; 'Y'; 'Z']  outPortNames=['v'; 'c'; '0'; '1'; '2'; '3'; '4'; '5'; '6'; '7'; '8'; '9'; 'A'; 'B'; 'D'; 'E'; 'F'; 'G'; 'H'; 'I'; 'J'; 'K'; 'L'; 'M'; 'N'; 'O'; 'P'; 'Q'; 'R'; 'S'; 'T'; 'U'; 'W'; 'X'; 'Y'; 'Z']  dspbaimage=dspba_prim.jpg  text=fprintf('In');  style=Optimised  dataSignals=1  foldingEnabled=off  channels=1  sampleRate=200  packetBeginPresent=off  packetBeginEnabled=off  visibilities=dspba_ChannelInVis(gcb)  latencyCorrection=0  version=20141013
  ChannelOut : DSPBAPrim/ChannelOut  primtype=channelout  nInputs=dspba_internal_get_channel_ports(gcb)  nOutputs=dspba_internal_get_channel_ports(gcb)  omode=Inherit via internal rule  otype=sfix(16)  scale=2^-15  rndmethod=Unbiased  factor=1  satmethod=Symmetric  shift_vec=[0 1 2 -1]  value=3  inPortNames=['v'; 'c'; '0'; '1'; '2'; '3'; '4'; '5'; '6'; '7'; '8'; '9'; 'A'; 'B'; 'D'; 'E'; 'F'; 'G'; 'H'; 'I'; 'J'; 'K'; 'L'; 'M'; 'N'; 'O'; 'P'; 'Q'; 'R'; 'S'; 'T'; 'U'; 'W'; 'X'; 'Y'; 'Z']  outPortNames=['v'; 'c'; '0'; '1'; '2'; '3'; '4'; '5'; '6'; '7'; '8'; '9'; 'A'; 'B'; 'D'; 'E'; 'F'; 'G'; 'H'; 'I'; 'J'; 'K'; 'L'; 'M'; 'N'; 'O'; 'P'; 'Q'; 'R'; 'S'; 'T'; 'U'; 'W'; 'X'; 'Y'; 'Z']  dspbaimage=dspba_prim.jpg  text=fprintf('Out%s', AdvDSPBChannelOutDisplay(latency));  style=Optimised  dataSignals=3  foldingEnabled=off  channels=1  sampleRate=200  packetBeginPresent=off  packetBeginEnabled=off  visibilities=dspba_ChannelOutVis(gcb)  latency=24  latencyCorrection=0  version=20141013
  ScalFact : Subsystem
  SynthesisInfo : DSPBAPrim/SynthesisInfo  primtype=synthinfo  nInputs=0  nOutputs=0  omode=Inherit via internal rule  otype=sfix(16)  scale=2^-15  rndmethod=Truncate  factor=1  satmethod=Symmetric  shift_vec=[0 1 2 -1]  value=99  inPortNames=[' '; ' ';]  outPortNames=[' ']  dspbaimage=dspba_prim.jpg  text=fprintf('Style=%s', style);  style=Scheduled  visibilities=32768  constraintInUse=off  constraintRelation=>  constraintLimit=50  bitAccurate=off  version=20150220
  qv : Outport
  qc : Outport  Port=2
  Out_c : Outport  Port=3
  count_o : Outport  Port=4
  sig_i : Outport  Port=5
  wires:
  v/1 -> ChannelIn/1
  c/1 -> ChannelIn/2
  ScalFact/1(qv) -> ChannelOut/1
  ScalFact/2(qc) -> ChannelOut/2
  ScalFact/3(Out_c) -> ChannelOut/3
  d/1 -> ChannelIn/3
  ChannelIn/1 -> ScalFact/1(v)
  ChannelIn/2 -> ScalFact/2(c)
  ChannelIn/3 -> ScalFact/3(d), ChannelOut/5
  ChannelOut/1 -> qv/1
  ChannelOut/2 -> qc/1
  ChannelOut/3 -> Out_c/1
  ScalFact/4(count_o) -> ChannelOut/4
  ChannelOut/4 -> count_o/1
  ChannelOut/5 -> sig_i/1

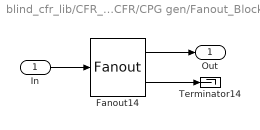
== system blind_cfr_lib/CFR_Block/CFR/CPG gen/Fanout_Block ==
  In : Inport
  Fanout14 : DSPBAPrim/Fanout  primtype=fanout  nInputs=1  nOutputs=evalAionMaskParam(gcb,'value',1)  omode=Inherit via internal rule  otype=sfix(16)  scale=2^-15  rndmethod=Unbiased  factor=1  satmethod=Symmetric  shift_vec=[0 1 2 -1]  value=2  inPortNames=[' '; ' ';]  outPortNames=[' ']  dspbaimage=dspba_prim.jpg  text=fprintf('fanout')  style=Optimised  visibilities=2^10+2^18  version=20150501  uninit=off
  Terminator14 : Terminator
  Out : Outport
  wires:
  Fanout14/2 -> Terminator14/1
  In/1 -> Fanout14/1
  Fanout14/1 -> Out/1

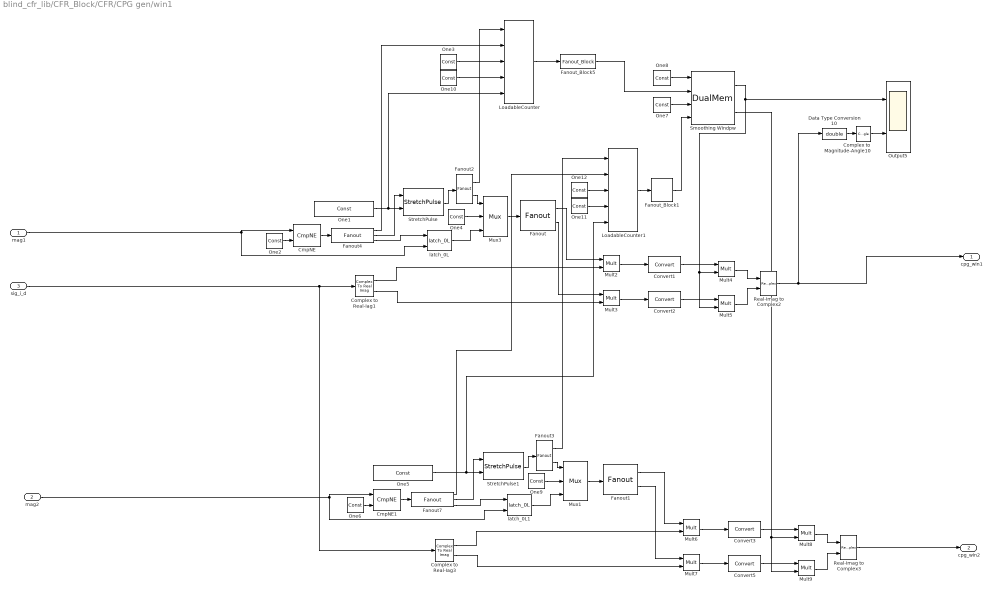
== system blind_cfr_lib/CFR_Block/CFR/CPG gen/win1 ==
  mag1 : Inport
  mag2 : Inport  Port=2
  sig_i_d : Inport  Port=3
  CmpNE : DSPBAPrim/CmpNE  primtype=cmpne  nInputs=2  nOutputs=1  omode=boolean  otype=sfix(16)  scale=2^-15  rndmethod=Unbiased  factor=1  satmethod=Symmetric  shift_vec=[0 1 2 -1]  value=0  inPortNames=[' '; ' ';]  outPortNames=[' ']  dspbaimage=dspba_prim.jpg  text=fprintf('~=');  style=Optimised  visibilities=0  advOptions=[]  version=20130117
  CmpNE1 : DSPBAPrim/CmpNE  primtype=cmpne  nInputs=2  nOutputs=1  omode=boolean  otype=sfix(16)  scale=2^-15  rndmethod=Unbiased  factor=1  satmethod=Symmetric  shift_vec=[0 1 2 -1]  value=0  inPortNames=[' '; ' ';]  outPortNames=[' ']  dspbaimage=dspba_prim.jpg  text=fprintf('~=');  style=Optimised  visibilities=0  advOptions=[]  version=20130117
  Complex to Magnitude-Angle10 : ComplexToMagnitudeAngle  Output=Magnitude
  Complex to Real-Iag1 : ComplexToRealImag
  Complex to Real-Iag3 : ComplexToRealImag
  Convert{1..3,5} (4 alike) : DSPBAPrim/Convert  primtype=convert  nInputs=1  nOutputs=1  omode=Specify via dialog  otype=sfix(16)  scale=2^-(15)  rndmethod=Unbiased  factor=1  satmethod=None  shift_vec=[0 1 2 -1]  value=round([0:255]/17)  inPortNames=[' '; ' ';]  outPortNames=[' '; 'c']  dspbaimage=dspba_prim.jpg  text=fprintf('convert');  style=Optimised  visibilities=8+64+256  clipdetect=off  floatPrecision=float32_m23  advOptions=[]  version=20130211
  Data Type Conversion10 : DataTypeConversion  OutDataTypeStr=double
  Fanout{,1..3} (4 alike) : DSPBAPrim/Fanout  primtype=fanout  nInputs=1  nOutputs=evalAionMaskParam(gcb,'value',1)  omode=Inherit via internal rule  otype=sfix(16)  scale=2^-15  rndmethod=Unbiased  factor=1  satmethod=Symmetric  shift_vec=[0 1 2 -1]  value=2  inPortNames=[' '; ' ';]  outPortNames=[' ']  dspbaimage=dspba_prim.jpg  text=fprintf('fanout')  style=Optimised  visibilities=2^10+2^18  version=20150501  uninit=off
  Fanout4 : DSPBAPrim/Fanout  primtype=fanout  nInputs=1  nOutputs=evalAionMaskParam(gcb,'value',1)  omode=Inherit via internal rule  otype=sfix(16)  scale=2^-15  rndmethod=Unbiased  factor=1  satmethod=Symmetric  shift_vec=[0 1 2 -1]  value=3  inPortNames=[' '; ' ';]  outPortNames=[' ']  dspbaimage=dspba_prim.jpg  text=fprintf('fanout')  style=Optimised  visibilities=2^10+2^18  version=20150501  uninit=off
  Fanout7 : DSPBAPrim/Fanout  primtype=fanout  nInputs=1  nOutputs=evalAionMaskParam(gcb,'value',1)  omode=Inherit via internal rule  otype=sfix(16)  scale=2^-15  rndmethod=Unbiased  factor=1  satmethod=Symmetric  shift_vec=[0 1 2 -1]  value=3  inPortNames=[' '; ' ';]  outPortNames=[' ']  dspbaimage=dspba_prim.jpg  text=fprintf('fanout')  style=Optimised  visibilities=2^10+2^18  version=20150501  uninit=off
  Fanout_Block1 : blind_cfr_lib/CFR_Block/CFR/CPG gen/Fanout_Block
  Fanout_Block5 : blind_cfr_lib/CFR_Block/CFR/CPG gen/Fanout_Block
  LoadableCounter : DSPBAPrim/LoadableCounter  primtype=loadablecounter  nInputs=5  nOutputs=1  omode=Inherit via internal rule  otype=ufix(16)  scale=2^-0  rndmethod=Unbiased  factor=1  satmethod=Symmetric  shift_vec=[0 1 2 -1]  value=[0 length(win) 1]  inPortNames=['en';'ld';'i ';'s ';'m ']  outPortNames=[' ']  dspbaimage=dspba_prim.jpg  text=fprintf('loadable\ncounter\n[%d %d %d]', value(1), value(2), value(3));  style=Optimised  visibilities=8 + 1024  version=20090407
  LoadableCounter1 : DSPBAPrim/LoadableCounter  primtype=loadablecounter  nInputs=5  nOutputs=1  omode=Inherit via internal rule  otype=ufix(16)  scale=2^-0  rndmethod=Unbiased  factor=1  satmethod=Symmetric  shift_vec=[0 1 2 -1]  value=[0 length(win) 1]  inPortNames=['en';'ld';'i ';'s ';'m ']  outPortNames=[' ']  dspbaimage=dspba_prim.jpg  text=fprintf('loadable\ncounter\n[%d %d %d]', value(1), value(2), value(3));  style=Optimised  visibilities=8 + 1024  version=20090407
  Mult{2..9} (8 alike) : DSPBAPrim/Mult  primtype=mult  nInputs=2  nOutputs=1  omode=Inherit via internal rule  otype=sfix(16)  scale=2^-15  rndmethod=Unbiased  factor=1  satmethod=Symmetric  shift_vec=[0 1 2 -1]  value=0  inPortNames=[' '; ' ';]  outPortNames=[' ']  dspbaimage=dspba_prim.jpg  text=fprintf('X');  style=Optimised  visibilities=8+2^18+2^19  floatPrecision=float32_m23  floatRounding=correct  advOptions=[]  version=20130115
  Mux1 : DSPBAPrim/Mux  primtype=mux  nInputs=evalAionMaskParam(gcb,'value',1)+1  nOutputs=1  omode=Inherit via internal rule  otype=sfix(16)  scale=2^-15  rndmethod=Unbiased  factor=1  satmethod=Symmetric  shift_vec=[0 1 2 -1]  value=2  inPortNames=['s'; 'd0'; 'd1'; 'd2'; 'd3'; 'd4'; 'd5'; 'd6'; 'd7'; 'd8'; 'd9';]  outPortNames=[' ']  dspbaimage=dspba_prim.jpg  text=fprintf('%s', primtype);  style=Optimised  visibilities=1032  version=20131025
  Mux3 : DSPBAPrim/Mux  primtype=mux  nInputs=evalAionMaskParam(gcb,'value',1)+1  nOutputs=1  omode=Inherit via internal rule  otype=sfix(16)  scale=2^-15  rndmethod=Unbiased  factor=1  satmethod=Symmetric  shift_vec=[0 1 2 -1]  value=2  inPortNames=['s'; 'd0'; 'd1'; 'd2'; 'd3'; 'd4'; 'd5'; 'd6'; 'd7'; 'd8'; 'd9';]  outPortNames=[' ']  dspbaimage=dspba_prim.jpg  text=fprintf('%s', primtype);  style=Optimised  visibilities=1032  version=20131025
  One1 : DSPBAPrim/Const  primtype=const  nInputs=0  nOutputs=1  omode=Specify via dialog  otype=uint(10)  scale=2^0  rndmethod=Unbiased  factor=1  satmethod=Symmetric  shift_vec=[0 1 2 -1]  value=Iter0_Param.winLen  inPortNames=['+'; '+';]  outPortNames=[' ']  dspbaimage=dspba_prim.jpg  text=fprintf('%s', num2str(value));  style=Optimised  visibilities=8 + 1024  floatPrecision=float32_m23  version=20120820
  One10 : DSPBAPrim/Const  primtype=const  nInputs=0  nOutputs=1  omode=Specify via dialog  otype=uint(10)  scale=2^0  rndmethod=Unbiased  factor=1  satmethod=Symmetric  shift_vec=[0 1 2 -1]  value=1  inPortNames=['+'; '+';]  outPortNames=[' ']  dspbaimage=dspba_prim.jpg  text=fprintf('%s', num2str(value));  style=Optimised  visibilities=8 + 1024  floatPrecision=float32_m23  version=20120820
  One11 : DSPBAPrim/Const  primtype=const  nInputs=0  nOutputs=1  omode=Specify via dialog  otype=uint(10)  scale=2^0  rndmethod=Unbiased  factor=1  satmethod=Symmetric  shift_vec=[0 1 2 -1]  value=1  inPortNames=['+'; '+';]  outPortNames=[' ']  dspbaimage=dspba_prim.jpg  text=fprintf('%s', num2str(value));  style=Optimised  visibilities=8 + 1024  floatPrecision=float32_m23  version=20120820
  One12 : DSPBAPrim/Const  primtype=const  nInputs=0  nOutputs=1  omode=Specify via dialog  otype=uint(10)  scale=2^0  rndmethod=Unbiased  factor=1  satmethod=Symmetric  shift_vec=[0 1 2 -1]  value=0  inPortNames=['+'; '+';]  outPortNames=[' ']  dspbaimage=dspba_prim.jpg  text=fprintf('%s', num2str(value));  style=Optimised  visibilities=8 + 1024  floatPrecision=float32_m23  version=20120820
  One2 : DSPBAPrim/Const  primtype=const  nInputs=0  nOutputs=1  omode=Inherit via internal rule  otype=sfix(16)  scale=2^-15  rndmethod=Unbiased  factor=1  satmethod=Symmetric  shift_vec=[0 1 2 -1]  value=0  inPortNames=['+'; '+';]  outPortNames=[' ']  dspbaimage=dspba_prim.jpg  text=fprintf('%s', num2str(value));  style=Optimised  visibilities=8 + 1024  floatPrecision=float32_m23  version=20120820
  One3 : DSPBAPrim/Const  primtype=const  nInputs=0  nOutputs=1  omode=Specify via dialog  otype=uint(10)  scale=2^0  rndmethod=Unbiased  factor=1  satmethod=Symmetric  shift_vec=[0 1 2 -1]  value=0  inPortNames=['+'; '+';]  outPortNames=[' ']  dspbaimage=dspba_prim.jpg  text=fprintf('%s', num2str(value));  style=Optimised  visibilities=8 + 1024  floatPrecision=float32_m23  version=20120820
  One4 : DSPBAPrim/Const  primtype=const  nInputs=0  nOutputs=1  omode=Specify via dialog  otype=ufix(16)  scale=2^-15  rndmethod=Unbiased  factor=1  satmethod=Symmetric  shift_vec=[0 1 2 -1]  value=0  inPortNames=['+'; '+';]  outPortNames=[' ']  dspbaimage=dspba_prim.jpg  text=fprintf('%s', num2str(value));  style=Optimised  visibilities=8 + 1024  floatPrecision=float32_m23  version=20120820
  One5 : DSPBAPrim/Const  primtype=const  nInputs=0  nOutputs=1  omode=Specify via dialog  otype=uint(10)  scale=2^0  rndmethod=Unbiased  factor=1  satmethod=Symmetric  shift_vec=[0 1 2 -1]  value=Iter0_Param.winLen  inPortNames=['+'; '+';]  outPortNames=[' ']  dspbaimage=dspba_prim.jpg  text=fprintf('%s', num2str(value));  style=Optimised  visibilities=8 + 1024  floatPrecision=float32_m23  version=20120820
  One6 : DSPBAPrim/Const  primtype=const  nInputs=0  nOutputs=1  omode=Inherit via internal rule  otype=sfix(16)  scale=2^-15  rndmethod=Unbiased  factor=1  satmethod=Symmetric  shift_vec=[0 1 2 -1]  value=0  inPortNames=['+'; '+';]  outPortNames=[' ']  dspbaimage=dspba_prim.jpg  text=fprintf('%s', num2str(value));  style=Optimised  visibilities=8 + 1024  floatPrecision=float32_m23  version=20120820
  One7 : DSPBAPrim/Const  primtype=const  nInputs=0  nOutputs=1  omode=boolean  otype=sfix(16)  scale=2^-15  rndmethod=Unbiased  factor=1  satmethod=Symmetric  shift_vec=[0 1 2 -1]  value=0  inPortNames=['+'; '+';]  outPortNames=[' ']  dspbaimage=dspba_prim.jpg  text=fprintf('%s', num2str(value));  style=Optimised  visibilities=8 + 1024  floatPrecision=float32_m23  version=20120820
  One8 : DSPBAPrim/Const  primtype=const  nInputs=0  nOutputs=1  omode=Specify via dialog  otype=sfix(16)  scale=2^-15  rndmethod=Unbiased  factor=1  satmethod=Symmetric  shift_vec=[0 1 2 -1]  value=0  inPortNames=['+'; '+';]  outPortNames=[' ']  dspbaimage=dspba_prim.jpg  text=fprintf('%s', num2str(value));  style=Optimised  visibilities=8 + 1024  floatPrecision=float32_m23  version=20120820
  One9 : DSPBAPrim/Const  primtype=const  nInputs=0  nOutputs=1  omode=Specify via dialog  otype=ufix(16)  scale=2^-15  rndmethod=Unbiased  factor=1  satmethod=Symmetric  shift_vec=[0 1 2 -1]  value=0  inPortNames=['+'; '+';]  outPortNames=[' ']  dspbaimage=dspba_prim.jpg  text=fprintf('%s', num2str(value));  style=Optimised  visibilities=8 + 1024  floatPrecision=float32_m23  version=20120820
  Output5 : Scope  NumInputPorts=2
  Real-Imag to Complex2 : RealImagToComplex
  Real-Imag to Complex3 : RealImagToComplex
  Smoothing Windpw : DSPBAPrim/DualMem  primtype=dualmem  nInputs=4  nOutputs=2  omode=Inherit via internal rule  otype=sfix(16)  scale=2^-15  rndmethod=Unbiased  factor=1  satmethod=Symmetric  shift_vec=[0 1 2 -1]  value=fi(win,1,16,15)  inPortNames=['d1'; 'a1'; 'w1'; 'a2']  outPortNames=['q1'; 'q2']  dspbaimage=dspba_prim.jpg  text=fprintf('dmem%s',AdvDSPBDMemDisplay(UseDontCare));  style=Optimised  visibilities=8 + 1024 + 2^17  UseDontCare=on  TwinWritePorts=off  version=20141001
  StretchPulse : DSPBAControl/StretchPulse
  StretchPulse1 : DSPBAControl/StretchPulse
  latch_0L : DSPBAControl/latch_0L
  latch_0L1 : DSPBAControl/latch_0L
  cpg_win1 : Outport
  cpg_win2 : Outport  Port=2
  wires:
  Fanout1/2 -> Mult7/1
  Fanout1/1 -> Mult6/1
  Mux1/1 -> Fanout1/1
  Fanout/2 -> Mult3/1
  Fanout/1 -> Mult2/1
  Mux3/1 -> Fanout/1
  LoadableCounter1/1 -> Fanout_Block1/1
  One11/1 -> LoadableCounter1/4
  One12/1 -> LoadableCounter1/3
  One10/1 -> LoadableCounter/4
  One3/1 -> LoadableCounter/3
  Complex to Magnitude-Angle10/1 -> Output5/2
  Data Type Conversion10/1 -> Complex to Magnitude-Angle10/1
  latch_0L/1 -> Mux3/3
  One4/1 -> Mux3/2
  One2/1 -> CmpNE/2
  Convert1/1 -> Mult4/1
  Mult4/1 -> Real-Imag to Complex2/1
  Mult5/1 -> Real-Imag to Complex2/2
  Convert2/1 -> Mult5/1
  Real-Imag to Complex2/1 -> cpg_win1/1, Data Type Conversion10/1
  Smoothing Windpw/1 -> Output5/1, Mult4/2, Mult5/2
  One1/1 -> StretchPulse/2, LoadableCounter/5
  latch_0L1/1 -> Mux1/3
  One9/1 -> Mux1/2
  Smoothing Windpw/2 -> Mult8/2, Mult9/2
  Convert5/1 -> Mult9/1
  Mult6/1 -> Convert3/1
  Convert3/1 -> Mult8/1
  sig_i_d/1 -> Complex to Real-Iag1/1, Complex to Real-Iag3/1
  Mult8/1 -> Real-Imag to Complex3/1
  mag2/1 -> latch_0L1/2, CmpNE1/1
  Mult7/1 -> Convert5/1
  Mult9/1 -> Real-Imag to Complex3/2
  Complex to Real-Iag3/2 -> Mult7/2
  One5/1 -> StretchPulse1/2, LoadableCounter1/5
  One6/1 -> CmpNE1/2
  Complex to Real-Iag3/1 -> Mult6/2
  Complex to Real-Iag1/1 -> Mult2/2
  Mult2/1 -> Convert1/1
  Mult3/1 -> Convert2/1
  Complex to Real-Iag1/2 -> Mult3/2
  Real-Imag to Complex3/1 -> cpg_win2/1
  One7/1 -> Smoothing Windpw/3
  One8/1 -> Smoothing Windpw/1
  mag1/1 -> CmpNE/1, latch_0L/2
  Fanout2/2 -> Mux3/1
  StretchPulse/1 -> Fanout2/1
  Fanout2/1 -> LoadableCounter/1
  Fanout3/2 -> Mux1/1
  StretchPulse1/1 -> Fanout3/1
  Fanout3/1 -> LoadableCounter1/1
  Fanout_Block5/1 -> Smoothing Windpw/2
  Fanout_Block1/1 -> Smoothing Windpw/4
  CmpNE/1 -> Fanout4/1
  Fanout4/3 -> latch_0L/1
  Fanout4/2 -> StretchPulse/1
  Fanout4/1 -> LoadableCounter/2
  CmpNE1/1 -> Fanout7/1
  Fanout7/3 -> latch_0L1/1
  Fanout7/2 -> StretchPulse1/1
  Fanout7/1 -> LoadableCounter1/2
  LoadableCounter/1 -> Fanout_Block5/1
